simulink model "VD_SCE"  (R2024b)
settings: Solver=VariableStepAuto  StartTime=0.0  StopTime=10.0  RelTol=1e-3
settings Model: Creator=admin  LastModifiedBy=admin

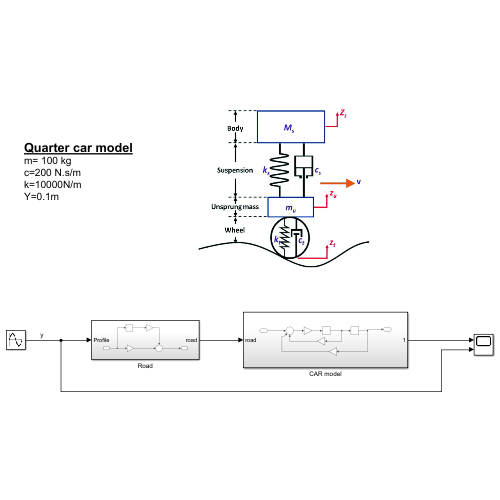
[thumbnail: Simulink's stored preview of the top-level diagram]
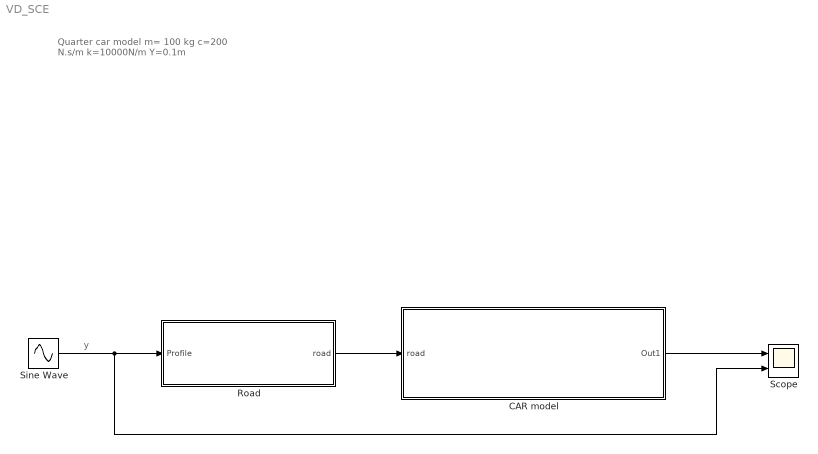
== system VD_SCE ==
  note: Quarter car model
      | m= 100 kg
      | c=200 N.s/m
      | k=10000N/m
      | Y=0.1m
  note: y
  CAR model : Subsystem
  Road : Subsystem
  Scope : Scope  NumInputPorts=2
  Sine Wave : Sin  Amplitude=0.1  Frequency=0.5  SampleTime=0
  wires:
  Sine Wave/1 -> Road/1(Profile), Scope/2
  CAR model/1(Out1) -> Scope/1
  Road/1(road) -> CAR model/1(road)

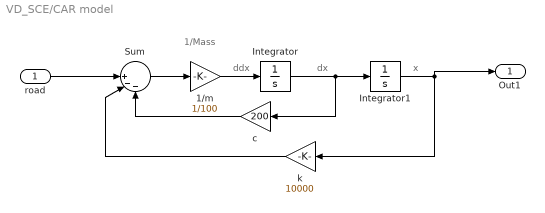
== system VD_SCE/CAR model ==
  note: 1/Mass
  note: x
  note: dx
  note: ddx
  road : Inport
  1/m : Gain  Gain=1/100
  Integrator : Integrator
  Integrator1 : Integrator
  Sum : Sum  Inputs=||+--
  c : Gain  Gain=200
  k : Gain  Gain=10000
  Out1 : Outport
  wires:
  road/1 -> Sum/1
  Integrator1/1 -> Out1/1, k/1
  Sum/1 -> 1/m/1
  Integrator/1 -> c/1, Integrator1/1
  k/1 -> Sum/2
  1/m/1 -> Integrator/1
  c/1 -> Sum/3

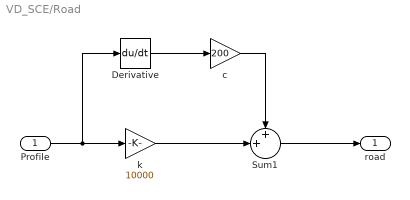
== system VD_SCE/Road ==
  Profile : Inport
  " c" : Gain  Gain=200
  " k" : Gain  Gain=10000
  Derivative : Derivative
  Sum1 : Sum  Inputs=++|
  road : Outport
  wires:
  Profile/1 -> Derivative/1, " k"/1
  " c"/1 -> Sum1/1
  Derivative/1 -> " c"/1
  " k"/1 -> Sum1/2
  Sum1/1 -> road/1
